simulink model "Test_Manual_Timer_16bit"  (R2023a)
settings: Solver=VariableStepAuto  StartTime=0.0  StopTime=inf  RelTol=1e-3  EnableMultiTasking=on
libraries: simulink_extras x3, Miscellaneous x3, Counters_Lib x2, Memory_Blocks_Lib x2, Decoders_Lib x1, Word_Multiplexers_Lib x1
settings Model: PacingRate=11  Creator=Jozko Mrkvicka  LastModifiedBy=Jozko Mrkvicka
settings SolverCC: AlgebraicLoopSolver=TrustRegion
settings DataIOCC: ReturnWorkspaceOutputs=off
settings OptimizationCC: LifeSpan=inf
settings DebuggingCC: UnconnectedInputMsg=warning  UnconnectedOutputMsg=warning  UnconnectedLineMsg=warning  SFUnexpectedBacktrackingDiag=warning  SFNoUnconditionalDefaultTransitionDiag=warning  ArithmeticOperatorsInVariantConditions=warning
settings ModelReferenceCC: EnableRefExpFcnMdlSchedulingChecks=on
settings SFSimCC: SimUseLocalCustomCode=off  CustomCodeUndefinedFunction=UseInterfaceOnly
settings RTWCC: RTWUseLocalCustomCode=off
settings CodeAppCC: StateflowObjectComments=on
settings GRTTargetCC: TargetLangStandard=C89/C90 (ANSI)
settings ConfigComp: CovMetricSettings=dw  CovSaveCumulativeToWorkspaceVar=on  CovSaveSingleToWorkspaceVar=on  CovExternalEMLEnable=off
settings SimscapeCC: SimscapeNormalizeSystem=off

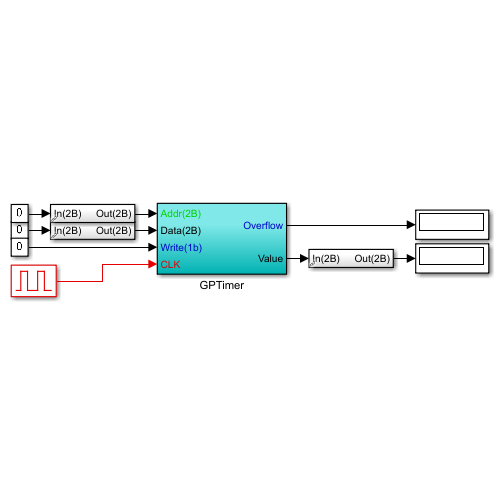
[thumbnail: Simulink's stored preview of the top-level diagram]
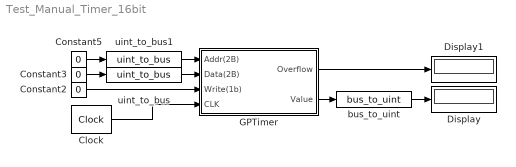
== system Test_Manual_Timer_16bit ==
  Clock : simulink_extras/Flip Flops/Clock  period=1
  Constant2 : Constant  Value=0  OutDataTypeStr=boolean
  Constant3 : Constant  Value=0  OutDataTypeStr=uint16
  Constant5 : Constant  Value=0  OutDataTypeStr=uint16
  Display : Display
  Display1 : Display
  GPTimer : Subsystem
  bus_to_uint : Miscellaneous/bus_to_uint  SystemSampleTime=-1  VariantActivationTime=update diagram  Latency=0  AutoFrameSizeCalculation=off
  uint_to_bus : Miscellaneous/uint_to_bus  SystemSampleTime=-1  VariantActivationTime=update diagram  Latency=0  AutoFrameSizeCalculation=off
  uint_to_bus1 : Miscellaneous/uint_to_bus  SystemSampleTime=-1  VariantActivationTime=update diagram  Latency=0  AutoFrameSizeCalculation=off
  wires:
  bus_to_uint/1 -> Display/1
  GPTimer/2(Value) -> bus_to_uint/1
  GPTimer/1(Overflow) -> Display1/1
  Constant3/1 -> uint_to_bus/1
  Constant5/1 -> uint_to_bus1/1
  uint_to_bus1/1 -> GPTimer/1(Addr(2B))
  uint_to_bus/1 -> GPTimer/2(Data(2B))
  Clock/1 -> GPTimer/4(CLK)
  Constant2/1 -> GPTimer/3(Write(1b))

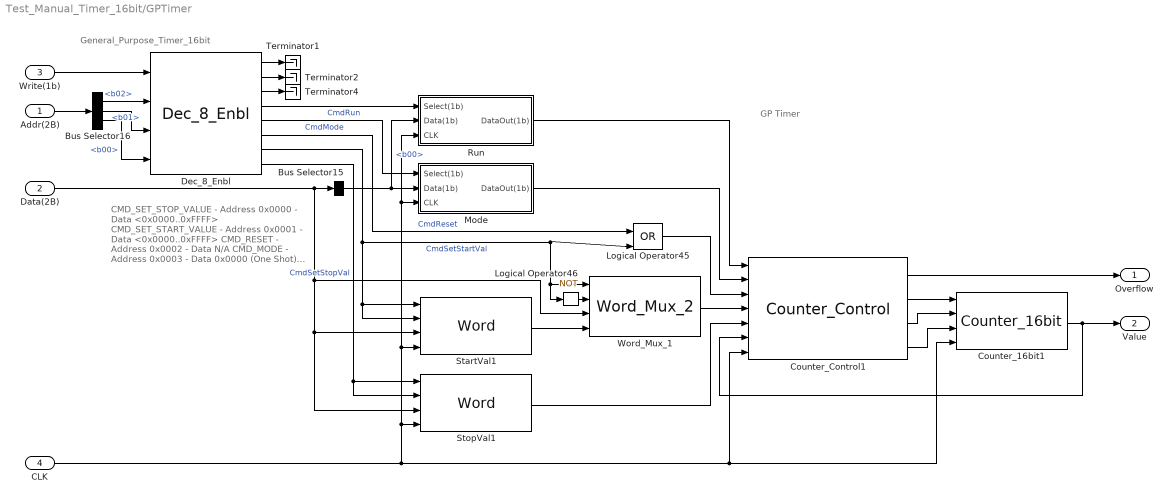
== system Test_Manual_Timer_16bit/GPTimer ==
  note: GP Timer
  note: General_Purpose_Timer_16bit
  note: CMD_SET_STOP_VALUE
      | - Address 0x0000
      | - Data   <0x0000..0xFFFF>
      |
      | CMD_SET_START_VALUE
      | - Address 0x0001
      | - Data   <0x0000..0xFFFF>
      |
      | CMD_RESET
      | - Address 0x0002
      | - Data    N/A
      |
      | CMD_MODE
      | - Address 0x0003
      | - Data    0x0000 (One Shot)
      |           0x0001 (Free Run)
      |
      | CMD_RUN
      | - Address 0x0004
      | - Data    0x0000 (Halt)
      |           0x0001 (Run)
  Addr(2B) : Inport
  Data(2B) : Inport  Port=2
  Write(1b) : Inport  Port=3
  CLK : Inport  Port=4
  Bus Selector15 : BusSelector  OutputSignals=b00
  Bus Selector16 : BusSelector  OutputSignals=b02,b01,b00
  Counter_16bit1 : Counters_Lib/Counter_16bit  SystemSampleTime=-1  VariantActivationTime=update diagram  Latency=0  AutoFrameSizeCalculation=off
  Counter_Control1 : Counters_Lib/Counter_Control  SystemSampleTime=-1  VariantActivationTime=update diagram  Latency=0  AutoFrameSizeCalculation=off
  Dec_8_Enbl : Decoders_Lib/Dec_8_Enbl  SystemSampleTime=-1  VariantActivationTime=update diagram  Latency=0  AutoFrameSizeCalculation=off
  Logical Operator45 : Logic  Operator=OR  IconShape=distinctive  AllPortsSameDT=off  OutDataTypeStr=boolean
  Logical Operator46 : Logic  Operator=NOT  Inputs=4  IconShape=distinctive  AllPortsSameDT=off  OutDataTypeStr=boolean
  Mode : Subsystem  AncestorBlock=Memory_Blocks_Lib/Bit
      settings: LibrarySourceBlock=Memory_Blocks_Lib/Bit
  Run : Subsystem  AncestorBlock=Memory_Blocks_Lib/Bit
      settings: LibrarySourceBlock=Memory_Blocks_Lib/Bit
  StartVal1 : Memory_Blocks_Lib/Word  SystemSampleTime=-1  VariantActivationTime=update diagram  Latency=0  AutoFrameSizeCalculation=off
  StopVal1 : Memory_Blocks_Lib/Word  SystemSampleTime=-1  VariantActivationTime=update diagram  Latency=0  AutoFrameSizeCalculation=off
  Terminator1 : Terminator
  Terminator2 : Terminator
  Terminator4 : Terminator
  Word_Mux_1 : Word_Multiplexers_Lib/Word_Mux_2  SystemSampleTime=-1  VariantActivationTime=update diagram  Latency=0  AutoFrameSizeCalculation=off
  Overflow : Outport
  Value : Outport  Port=2
  wires:
  Dec_8_Enbl/3 -> Terminator4/1
  Bus Selector16/1 -> Dec_8_Enbl/2  "<b02>"
  Counter_Control1/4 -> Counter_16bit1/3
  Dec_8_Enbl/4 -> Run/1(Select(1b))  "CmdRun"
  StopVal1/1 -> Counter_Control1/5
  Dec_8_Enbl/7 -> StartVal1/2, StartVal1/1, Logical Operator46/1, Word_Mux_1/1, Logical Operator45/2  "CmdSetStartVal"
  Counter_Control1/3 -> Counter_16bit1/2
  Data(2B)/1 -> StopVal1/3, StartVal1/3, Word_Mux_1/3, Bus Selector15/1
  Dec_8_Enbl/8 -> StopVal1/2, StopVal1/1  "CmdSetStopVal"
  Bus Selector16/3 -> Dec_8_Enbl/4  "<b00>"
  Counter_Control1/2 -> Counter_16bit1/1
  StartVal1/1 -> Word_Mux_1/4
  Run/1(DataOut(1b)) -> Counter_Control1/1
  Dec_8_Enbl/6 -> Logical Operator45/1  "CmdReset"
  Mode/1(DataOut(1b)) -> Counter_Control1/2
  Word_Mux_1/1 -> Counter_Control1/4
  Bus Selector16/2 -> Dec_8_Enbl/3  "<b01>"
  Counter_16bit1/1 -> Counter_Control1/6, Value/1
  Dec_8_Enbl/5 -> Mode/1(Select(1b))  "CmdMode"
  CLK/1 -> StartVal1/4, Mode/3(CLK), Run/3(CLK), StopVal1/4, Counter_16bit1/4, Counter_Control1/7
  Logical Operator45/1 -> Counter_Control1/3
  Logical Operator46/1 -> Word_Mux_1/2
  Bus Selector15/1 -> Mode/2(Data(1b)), Run/2(Data(1b))  "<b00>"
  Dec_8_Enbl/2 -> Terminator2/1
  Dec_8_Enbl/1 -> Terminator1/1
  Counter_Control1/1 -> Overflow/1
  Addr(2B)/1 -> Bus Selector16/1
  Write(1b)/1 -> Dec_8_Enbl/1

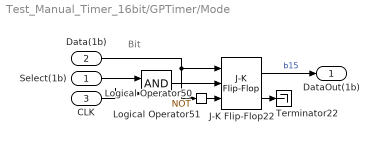
== system Test_Manual_Timer_16bit/GPTimer/Mode ==
  note: Bit
  Select(1b) : Inport  OutDataTypeStr=boolean
  Data(1b) : Inport  Port=2  OutDataTypeStr=boolean
  CLK : Inport  Port=3
  J-K Flip-Flop22 : simulink_extras/Flip Flops/J-K Flip-Flop  initial_condition=0
  Logical Operator50 : Logic  Operator=NOT  IconShape=distinctive  AllPortsSameDT=off  OutDataTypeStr=boolean
  Logical Operator51 : Logic  IconShape=distinctive  AllPortsSameDT=off  OutDataTypeStr=boolean
  Terminator22 : Terminator
  DataOut(1b) : Outport
  wires:
  Logical Operator51/1 -> J-K Flip-Flop22/2
  J-K Flip-Flop22/1 -> DataOut(1b)/1  "b15"
  J-K Flip-Flop22/2 -> Terminator22/1
  Data(1b)/1 -> J-K Flip-Flop22/1, Logical Operator50/1
  CLK/1 -> Logical Operator51/2
  Logical Operator50/1 -> J-K Flip-Flop22/3
  Select(1b)/1 -> Logical Operator51/1

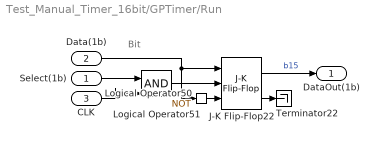
== system Test_Manual_Timer_16bit/GPTimer/Run ==
  note: Bit
  Select(1b) : Inport  OutDataTypeStr=boolean
  Data(1b) : Inport  Port=2  OutDataTypeStr=boolean
  CLK : Inport  Port=3
  J-K Flip-Flop22 : simulink_extras/Flip Flops/J-K Flip-Flop  initial_condition=0
  Logical Operator50 : Logic  Operator=NOT  IconShape=distinctive  AllPortsSameDT=off  OutDataTypeStr=boolean
  Logical Operator51 : Logic  IconShape=distinctive  AllPortsSameDT=off  OutDataTypeStr=boolean
  Terminator22 : Terminator
  DataOut(1b) : Outport
  wires:
  Logical Operator51/1 -> J-K Flip-Flop22/2
  J-K Flip-Flop22/1 -> DataOut(1b)/1  "b15"
  J-K Flip-Flop22/2 -> Terminator22/1
  Data(1b)/1 -> J-K Flip-Flop22/1, Logical Operator50/1
  CLK/1 -> Logical Operator51/2
  Logical Operator50/1 -> J-K Flip-Flop22/3
  Select(1b)/1 -> Logical Operator51/1
